simulink model "system_id_simulink"  (R2025a)
settings: Solver=VariableStepAuto  StartTime=0.0  StopTime=1  FixedStep=0.05  RelTol=1e-3
values from neighbouring files (symbols this model uses):
  w = W(i)    [noisy_id.m]
undefined symbols (not defined in the file or in its folder): use_pade
settings Model: Creator=DELL  LastModifiedBy=USER

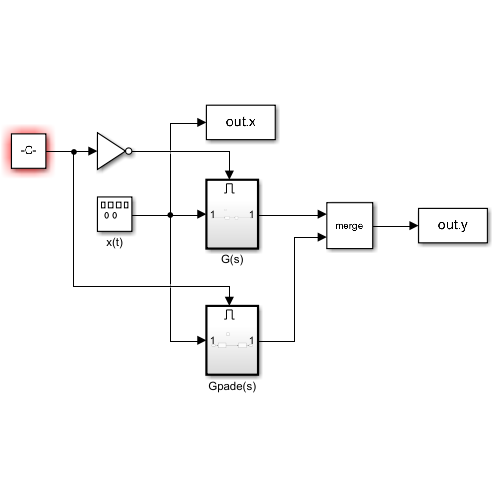
[thumbnail: Simulink's stored preview of the top-level diagram]
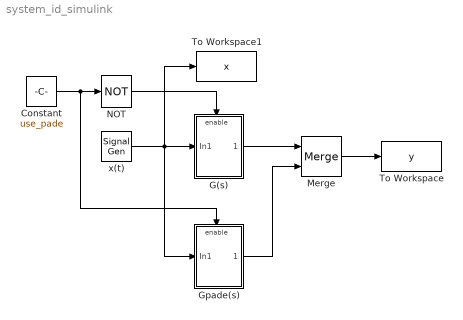
== system system_id_simulink ==
  Constant : Constant  Value=use_pade
  G(s) : Subsystem
  Gpade(s) : Subsystem
  Merge : Merge
  NOT : Logic  Operator=NOT  IconShape=distinctive  AllPortsSameDT=off  OutDataTypeStr=boolean
  To Workspace : ToWorkspace  VariableName=y  SaveFormat=Timeseries  SampleTime=-1
  To Workspace1 : ToWorkspace  VariableName=x  SaveFormat=Timeseries  SampleTime=-1
  x(t) : SignalGenerator  Frequency=w  Units=rad/sec
  wires:
  x(t)/1 -> Gpade(s)/1(In1), G(s)/1(In1), To Workspace1/1
  Constant/1 -> Gpade(s)/Enable, NOT/1
  G(s)/1(Out1) -> Merge/1
  NOT/1 -> G(s)/Enable
  Gpade(s)/1(Out1) -> Merge/2
  Merge/1 -> To Workspace/1

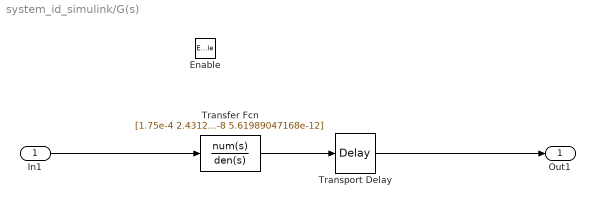
== system system_id_simulink/G(s) ==
  In1 : Inport
  Enable : EnablePort
  Transfer Fcn : TransferFcn  Numerator=[1.75e-4 2.431275e-7 9.284625e-12]  Denominator=[1 3.87704e-2 2.551212584e-4 8.784303992e-8 5.61989047168e-12]
  Transport Delay : TransportDelay  DelayTime=9.3  BufferSize=2048
  Out1 : Outport
  wires:
  Transfer Fcn/1 -> Transport Delay/1
  Transport Delay/1 -> Out1/1
  In1/1 -> Transfer Fcn/1

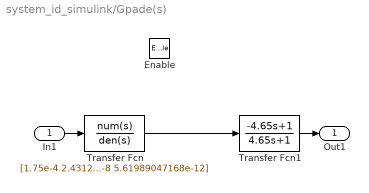
== system system_id_simulink/Gpade(s) ==
  In1 : Inport
  Enable : EnablePort
  Transfer Fcn : TransferFcn  Numerator=[1.75e-4 2.431275e-7 9.284625e-12]  Denominator=[1 3.87704e-2 2.551212584e-4 8.784303992e-8 5.61989047168e-12]
  Transfer Fcn1 : TransferFcn  Numerator=[-4.65 1]  Denominator=[4.65 1]
  Out1 : Outport
  wires:
  Transfer Fcn/1 -> Transfer Fcn1/1
  In1/1 -> Transfer Fcn/1
  Transfer Fcn1/1 -> Out1/1
